simulink model "mod10"  (R2018b)
settings: Solver=FixedStepAuto  StartTime=0.0  StopTime=200  FixedStep=1e-2  RelTol=1e-3  EnableMultiTasking=on
values from neighbouring files (symbols this model uses):
  h = 4    [mod1s.m]
  K = 19    [mod1s.m]
  k1 = 3    [mod1s.m]
  k2 = 40    [mod1s.m]
  T = 29    [mod1s.m]
  x0 = -100    [mod1s.m]
  y0 = 0    [mod1s.m]
libraries: simulink_extras x1
settings Model: Creator=user  LastModifiedBy=ogure
settings SolverCC: SolverResetMethod=Robust
settings DataIOCC: LimitDataPoints=on  SaveFormat=Array  SaveOutput=off  OutputSaveName=X,X4,L,H
settings OptimizationCC: LifeSpan=inf
settings DebuggingCC: SolverPrmCheckMsg=warning  SFUnexpectedBacktrackingDiag=warning  SFNoUnconditionalDefaultTransitionDiag=warning  SFExecutionAtInitializationDiag=none
settings HardwareCC: ProdBitPerPointer=32  ProdBitPerSizeT=32  ProdBitPerPtrDiffT=32  ProdLargestAtomicFloat=None  ProdIntDivRoundTo=Undefined  ProdEndianess=Unspecified  ProdWordSize=32  ProdHWDeviceType=32-bit Generic
settings ModelReferenceCC: PropagateSignalLabelsOutOfModel=off
settings SFSimCC: SimUseLocalCustomCode=off
settings RTWCC: RTWUseLocalCustomCode=off
settings CodeAppCC: StateflowObjectComments=on
settings GRTTargetCC: TargetLangStandard=C89/C90 (ANSI)  GeneratePreprocessorConditionals=Disable all
settings ConfigComp: CovMetricSettings=dw  CovHtmlReporting=on  CovSaveCumulativeToWorkspaceVar=on  CovSaveSingleToWorkspaceVar=on  CovExternalEMLEnable=off  CovSFcnEnable=off

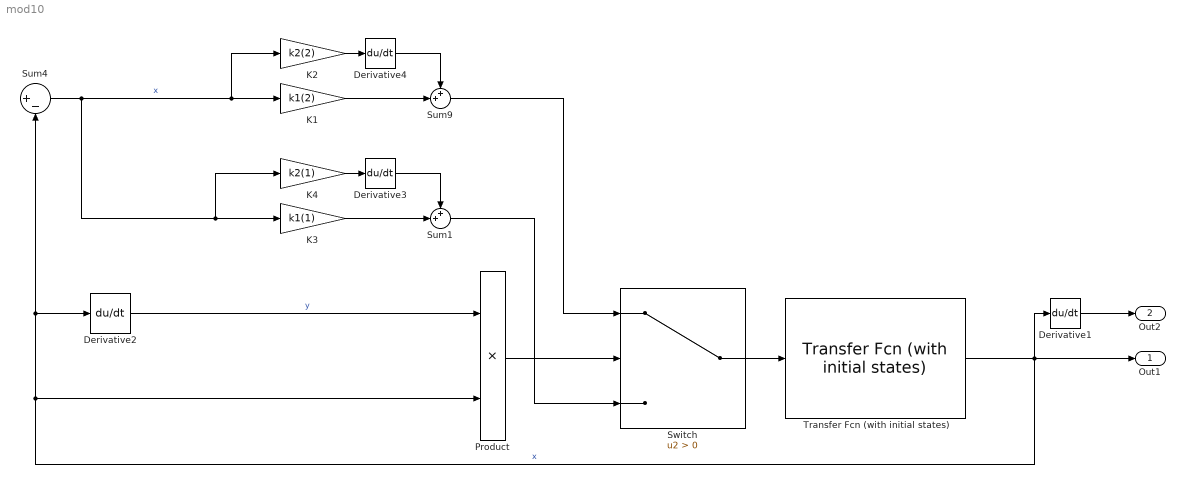
== system mod10 ==
  Derivative{1..4} (4 alike) : Derivative  CoefficientInTFapproximation=0.00000001
  K1 : Gain  Gain=k1(2)
  K2 : Gain  Gain=k2(2)
  K3 : Gain  Gain=k1(1)
  K4 : Gain  Gain=k2(1)
  Product : Product
  Sum1 : Sum  Inputs=++|
  Sum4 : Sum  Inputs=|+-
  Sum9 : Sum  Inputs=++|
  Switch : Switch  Criteria=u2 > Threshold  ZeroCross=off
  Transfer Fcn (with initial states) : simulink_extras/Additional Linear/Transfer Fcn (with initial states)  N=[K]  D="[ T^2  2*T*h  1]"  X0=[x0, y0]
  Out1 : Outport  SignalName=x
  Out2 : Outport  Port=2  SignalName=y
  wires:
  Switch/1 -> Transfer Fcn (with initial states)/1
  Derivative2/1 -> Product/1  "y"
  Product/1 -> Switch/2
  Derivative1/1 -> Out2/1
  Transfer Fcn (with initial states)/1 -> Derivative1/1, Product/2, Sum4/2, Derivative2/1, Out1/1  "x"
  K1/1 -> Sum9/2
  K2/1 -> Derivative4/1
  Derivative4/1 -> Sum9/1
  Sum9/1 -> Switch/1
  K4/1 -> Derivative3/1
  Derivative3/1 -> Sum1/1
  K3/1 -> Sum1/2
  Sum4/1 -> K4/1, K3/1, K1/1, K2/1  "x"
  Sum1/1 -> Switch/3
